simulink model "Generator_Testrig"  (R2019b)
settings: Solver=ode23t  StartTime=0.0  StopTime=15  MaxStep=0.01  RelTol=1e-5  EnableMultiTasking=on
PreLoadFcn:
  | load Generator_Test_DATA
PostLoadFcn:
  | warning off ne_sli:simulator:input:FilteredInputs
undefined symbols (not defined in the file): radps2rpm, WT_Params
libraries: powerlib x6, fl_lib x6, nesl_utility x4, Generator_Lib x1, powerlib_extras x1, Geartrain_Lib x1, simulink x1
Description:
  | Copyright 2009-2017 The MathWorks, Inc. MathWorks, Inc.
settings Model: Creator=smiller  LastModifiedBy=bhisma
settings DataIOCC: LimitDataPoints=on  SaveFormat=Array  SignalLoggingSaveFormat=ModelDataLogs  ReturnWorkspaceOutputs=off
settings OptimizationCC: ExpressionDepthLimit=2147483647  LifeSpan=inf
settings DebuggingCC: UnderspecifiedInitializationDetection=Classic  MergeDetectMultiDrivingBlocksExec=none  SolverPrmCheckMsg=warning  FcnCallInpInsideContextMsg=warning  AllowSymbolicDim=off  StateNameClashWarn=warning  SFUnexpectedBacktrackingDiag=warning  SFNoUnconditionalDefaultTransitionDiag=warning  SFExecutionAtInitializationDiag=none  ArithmeticOperatorsInVariantConditions=warning
settings HardwareCC: ProdBitPerPointer=32  ProdBitPerSizeT=32  ProdBitPerPtrDiffT=32  ProdLargestAtomicFloat=None  ProdIntDivRoundTo=Undefined  ProdEndianess=Unspecified  ProdWordSize=32  ProdHWDeviceType=32-bit Generic
settings ModelReferenceCC: PropagateSignalLabelsOutOfModel=off
settings SFSimCC: SimUseLocalCustomCode=off  CustomCodeUndefinedFunction=UseInterfaceOnly
settings RTWCC: RTWUseLocalCustomCode=off
settings CodeAppCC: StateflowObjectComments=on
settings GRTTargetCC: TargetLangStandard=C89/C90 (ANSI)  GeneratePreprocessorConditionals=Disable all  CombineOutputUpdateFcns=off  GRTInterface=on
settings ConfigComp: CovMetricSettings=dw  CovHtmlReporting=on  CovSaveCumulativeToWorkspaceVar=on  CovSaveSingleToWorkspaceVar=on  CovExternalEMLEnable=off  CovSFcnEnable=off
settings SimscapeCC: SimscapeNormalizeSystem=off  SimscapeNominalValues="[{\"value\":\"10\",\"unit\":\"V\"},{\"value\":\"1\",\"unit\":\"A\"},{\"value\":\"10\",\"unit\":\"N*m\"},{\"value\":\"10\",\"unit\":\"bar\"},{\"value\":\"100\",\"unit\":\"kJ/kg\"},{\"value\":\"1\",\"unit\":\"kW\"},{\"value\":\"300\",\"unit\":\"K\"},{\"value\":\"100\",\"unit\":\"cm^3/s\"},{\"value\":\"1\",\"unit\":\"kN\"},{\"value\":\"1\",\"unit\":\"g/cm^3\"},{\"value\":\"1\",\"unit\":\"l\"},{\"value\":\"1\",\"unit\":\"cm^2\"},{\"value\":\"60\",\"unit\":\"Hz\"}]"

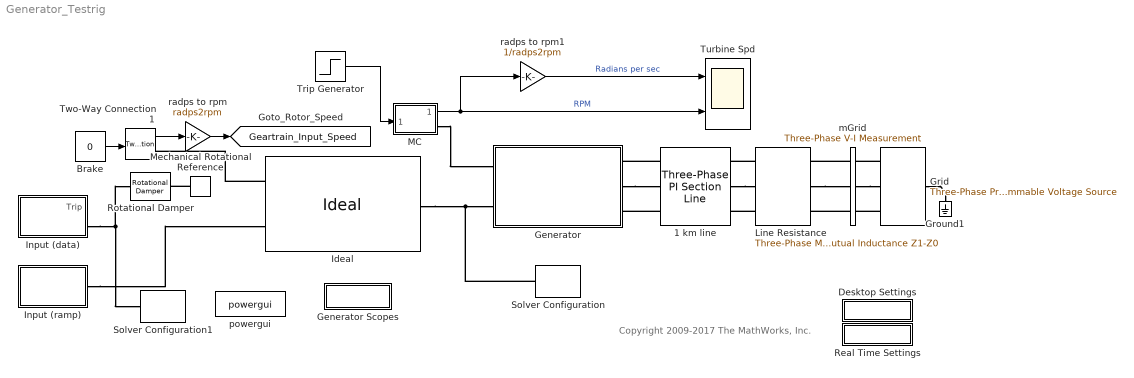
== system Generator_Testrig ==
  note: Copyright 2009-2017 The MathWorks, Inc.
  "1 km line " : powerlib/Elements/Three-Phase PI Section Line  LConnTagsString=a|b|c  RConnTagsString=A|B|C  Frequency=WT_Params.Grid.frequency  Resistances=[0.1153 0.413]  Inductances=[1.05e-3 3.32e-3]  Capacitances=[11.33e-009 5.01e-009]  Length=1
      settings: SourceProductName=Simscape Electrical
  Brake : Constant  Value=0
  Desktop Settings : Subsystem
      settings: OpenFcn=|
      | set_param(bdroot,'Solver','ODE23t','MaxStep','0.01');
      | 
      | tvar_solverBlock = find_system(bdroot, 'SubClassName', 'solver');
      | 
      | for i=1:size(tvar_solverBlock,1)
      | 
      | set_param(char(tvar_solverBlock(i)), 'UseLocalSolver','off','DoFixedCost','off');
      | end
      | 
      | clear tvar_solverBlock
      mask Display: disp('Desktop')
  Generator : Subsystem  BlockChoice=Full
      link override Full/B_Gen/Model/VI/Ia: GotoTag=tpdea4285c_d746_48d3_8c95_fd37d852a013_Ia
      link override Full/B_Gen/Model/VI/Ib: GotoTag=tpdea4285c_d746_48d3_8c95_fd37d852a013_Ib
      link override Full/B_Gen/Model/VI/Ic: GotoTag=tpdea4285c_d746_48d3_8c95_fd37d852a013_Ic
      link override Full/B_Gen/Model/VI/Va: GotoTag=tpdea4285c_d746_48d3_8c95_fd37d852a013_Va
      link override Full/B_Gen/Model/VI/Vb: GotoTag=tpdea4285c_d746_48d3_8c95_fd37d852a013_Vb
      link override Full/B_Gen/Model/VI/Vc: GotoTag=tpdea4285c_d746_48d3_8c95_fd37d852a013_Vc
      settings: AttributesFormatString=%<BlockChoice>  TemplateBlock=Generator_Lib/Generator  MemberBlocks=Full,Simple
      mask Display: disp(' ')
  Generator Scopes : Subsystem  AncestorBlock=Generator_Lib/Generator Scopes
  Grid : powerlib/Electrical Sources/Three-Phase Programmable Voltage Source  PositiveSequence=[WT_Params.Grid.voltage 0 WT_Params.Grid.frequency]  VariationEntity=None  VariationType=Table of time-amplitude pairs  VariationTypeAlt=Step  VariationStep=-0.15  VariationRate=10  VariationMagnitude=0.3  VariationFrequency=2  VariationTiming=[5 5.5]  VariationPhaseA=off  Amplitudes="[1.0  0.5  1.0 ]"  TimeValues="[0  10  10.1]"  HarmonicGeneration=off  HarmonicA=[1 -0.1 0 1]  HarmonicB=[2 0.15 35 2]  Timing="[5  5.5]"  BusType=swing  Pref=0  Qref=0  Qmin=-inf  Qmax=inf
      settings: SourceProductName=Simscape Electrical
  Ground1 : powerlib/Elements/Ground  LConnTagsString=a
      settings: SourceProductName=Simscape Electrical
  Ideal : Geartrain_Lib/Ideal  SystemSampleTime=-1
  Input (data) : Subsystem
  Input (ramp) : Subsystem  mask{start_speed=0, final_speed=14.3004, start_time=3, stop_time=10}
      mask prompts: start_speed "Start speed (rpm)"; final_speed "Final speed (rpm)"; start_time "Ramp start time"; stop_time "Ramp stop time"
  Line Resistance : powerlib/Elements/Three-Phase Mutual Inductance Z1-Z0  LConnTagsString=a|b|c  RConnTagsString=A|B|C  PositiveSequence="[0.1  1.0/(2*pi*60)]*WT_Params.Grid.voltage^2/2500e6"  ZeroSequence="[0.3  3.0/(2*pi*60)]*WT_Params.Grid.voltage^2/2500e6"
      settings: SourceProductName=Simscape Electrical  SourceProductBaseCode=PS
  MC : Subsystem
  Mechanical Rotational Reference : fl_lib/Mechanical/Rotational Elements/Mechanical Rotational Reference
  Real Time Settings : Subsystem
      settings: OpenFcn=|
      | tvar_Nonlinear_Iterations = '3';
      | tvar_StepSize = '0.001';
      | %tvar_LocalSolver='NE_TRAPEZOIDAL_ADVANCER';
      | tvar_LocalSolver='NE_BACKWARD_EULER_ADVANCER';
      | set_param(bdroot,'Solver','ode3','FixedStep','auto');
      | tvar_solverBlock = find_system(bdroot, 'SubClassName', 'solver');
      | for i=1:size(tvar_solverBlock,1)
      |     set_param(char(tvar_solverBlock(i)), 'UseLocalSolver','on','DoFixedCost','on','MaxNonlinIter',tvar_Nonlinear_Iterations,'LocalSolverChoice',tvar_LocalSolver,'LocalSolverSampleTime',tvar_StepSize);
      | end
      | clear tvar_Nonlinear_Iterations tvar_StepSize tvar_LocalSolver tvar_solverBlock
      mask Display: disp('Real Time')
  Rotational Damper : fl_lib/Mechanical/Rotational Elements/Rotational Damper  D=0.001 N*m/(rad/s)  w_specify=off  w_priority=High  w=0 rad/s  w_nominal_specify=off  w_nominal_unit=rad/s  w_nominal_value=1  t_specify=off  t_priority=High  t=0 N*m  t_nominal_specify=off  t_nominal_unit=N*m  t_nominal_value=1
  Solver Configuration : nesl_utility/Solver Configuration  PhysicalDomain=network_engine_domain  SubClassName=solver  LeftPortType=input  RightPortType=generic  Tones=[]  Harmonics=[]  SimulateNoise=off  Profile=off  UseLocalSampling=off  EnableSwitchedLinearOptims=on  FrequencyDomain=off  UseCCode=off  RelTol=0.001  AbsTol=1e-06  MinStep=1e-09  ToWorkspace=off  RevertToSquareIcSolve=off  NumHomotopyIterations=100  PhasorMode=off  PhasorModeNumHarmonics=1  DoDC=off  ResidualTolerance=1e-9  UseLocalSolver=off  LocalSolverChoice=NE_BACKWARD_EULER_ADVANCER  LocalSolverSampleTime=0.001  DoFixedCost=off  MaxNonlinIter=3  MaxModeIter=2  LinearAlgebra=Sparse  EquationFormulation=NE_TIME_EF  DelaysMemoryBudget=1024  AutomaticFiltering=on  FilteringTimeConstant=0.001  PartitionStorageMethod=AS_NEEDED  PartitionMemoryBudget=1024  PartitionMethod=FAST
  Solver Configuration1 : nesl_utility/Solver Configuration  PhysicalDomain=network_engine_domain  SubClassName=solver  LeftPortType=input  RightPortType=generic  Tones=[]  Harmonics=[]  SimulateNoise=off  Profile=off  UseLocalSampling=off  EnableSwitchedLinearOptims=on  FrequencyDomain=off  UseCCode=off  RelTol=0.001  AbsTol=1e-06  MinStep=1e-09  ToWorkspace=off  RevertToSquareIcSolve=off  NumHomotopyIterations=100  PhasorMode=off  PhasorModeNumHarmonics=1  DoDC=off  ResidualTolerance=1e-9  UseLocalSolver=off  LocalSolverChoice=NE_BACKWARD_EULER_ADVANCER  LocalSolverSampleTime=0.001  DoFixedCost=off  MaxNonlinIter=3  MaxModeIter=2  LinearAlgebra=Sparse  EquationFormulation=NE_TIME_EF  DelaysMemoryBudget=1024  AutomaticFiltering=on  FilteringTimeConstant=0.001  PartitionStorageMethod=AS_NEEDED  PartitionMemoryBudget=1024  PartitionMethod=FAST
  Trip Generator : Step  Time=10  Before=1  After=0  SampleTime=0
  Turbine Spd : Scope  NumInputPorts=2
  Two-Way Connection1 : TwoWayConnection
  mGrid : powerlib/Measurements/Three-Phase V-I Measurement  VoltageMeasurement=phase-to-ground  SetLabelV=on  LabelV=VmGrid  Vpu=on  VpuLL=off  CurrentMeasurement=no  SetLabelI=on  LabelI=ImGrid  Ipu=off  Pbase=1.5e6/0.9  Vbase=25e3  OutputType=Magnitude  PhasorSimulation=on  PSBequivalent=0
      settings: SourceProductName=Simscape Electrical
  powergui : powerlib/powergui  SimulationMode=Phasor  SampleTime=5e-6  frequency=60  Iterations=50  frequencyindice=60  Pbase=100e6  ErrMax=1e-4  UnitsV=kV  UnitsW=MW  buscounter=0  FunctionMessages=off  echomessages=off  EnableUseOfTLC=off  CurrentSourceSwitches=off  DisableSnubberDevices=off  DisableRonSwitches=off  DisableVfSwitches=off  DisplayEquations=off  AutomaticDiscreteSolvers=off  SolverType=Tustin  Interpol=off  ExternalGateDelay=off  methode=off  Ts=0  x0status=blocks  SPID=off  SwTol=0  HookPort=off  NonlinearTolerance=1e-4  nMaxIteration=100  ContinueOnMaxIteration=off  RestoreLinks=warning  ResistiveCurrentMeasurement=off  Frange=[0:2:500]  Ylog=off  Xlog=on  ShowGrid=off  save=off  variable=ZData  structure=0  ZoomFFT=on  StartTime=0.0  cycles=1  DisplayStyle=1  fundamental=60  FreqAxis=off  MaxFrequency=1000  frequencyindicesteady=1  RmsSteady=1  display=off
      settings: SourceProductName=Simscape Electrical
  radps to rpm : Gain  Gain=radps2rpm
  radps to rpm1 : Gain  Gain=1/radps2rpm
  tag scope: Geartrain_Input_Speed=global
  wires:
  MC/1(Speed) -> radps to rpm1/1, Turbine Spd/2  "RPM"
  Two-Way Connection1/1 -> radps to rpm/1
  Brake/1 -> Two-Way Connection1/1
  radps to rpm/1 -> [Geartrain_Input_Speed]
  radps to rpm1/1 -> Turbine Spd/1  "Radians per sec"
  Trip Generator/1 -> MC/1(Trip)
  connections:
  Grid/LConn1 -- Ground1/LConn1
  Line Resistance/RConn1 -- "1 km line "/LConn1
  "1 km line "/LConn2 -- Line Resistance/RConn2
  Line Resistance/RConn3 -- "1 km line "/LConn3
  Grid/RConn1 -- mGrid/LConn1
  mGrid/LConn2 -- Grid/RConn2
  Grid/RConn3 -- mGrid/LConn3
  mGrid/RConn1 -- Line Resistance/LConn1
  Line Resistance/LConn2 -- mGrid/RConn2
  mGrid/RConn3 -- Line Resistance/LConn3
  Ideal/RConn1 -- Solver Configuration/RConn1 -- Generator/LConn2
  "1 km line "/RConn1 -- Generator/RConn1
  Generator/RConn2 -- "1 km line "/RConn2
  "1 km line "/RConn3 -- Generator/RConn3
  MC/RConn1 -- Generator/LConn1
  Ideal/LConn1 -- Two-Way Connection1/RConn1
  Input (data)/RConn1 -- Solver Configuration1/RConn1 -- Rotational Damper/LConn1
  Input (ramp)/LConn1 -- Ideal/LConn2
  Mechanical Rotational Reference/LConn1 -- Rotational Damper/RConn1

== system Generator_Testrig/Desktop Settings ==

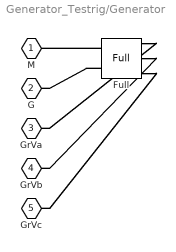
== system Generator_Testrig/Generator ==
  Full : Generator_Lib/Full  SystemSampleTime=-1
  M : PMIOPort  Side=Left
  G : PMIOPort  Port=2  Side=Left
  GrVa : PMIOPort  Port=3  Side=Right
  GrVb : PMIOPort  Port=4  Side=Right
  GrVc : PMIOPort  Port=5  Side=Right
  connections:
  Full/LConn1 -- M/RConn1
  Full/LConn2 -- G/RConn1
  Full/RConn1 -- GrVa/RConn1
  Full/RConn2 -- GrVb/RConn1
  Full/RConn3 -- GrVc/RConn1

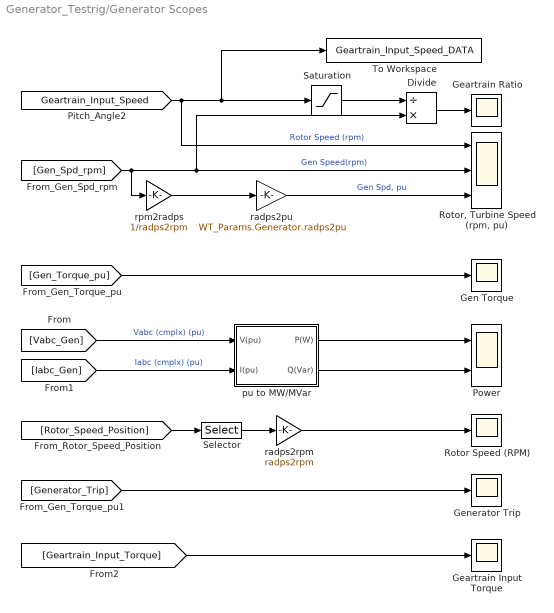
== system Generator_Testrig/Generator Scopes ==
  Divide : Product  Inputs=/*
  Geartrain Input Torque : Scope
  Geartrain Ratio : Scope
  Gen Torque : Scope
  Generator Trip : Scope
  Power : Scope  NumInputPorts=2
  Rotor Speed (RPM) : Scope
  "Rotor, Turbine Speed (rpm, pu)" : Scope  NumInputPorts=3
  Saturation : Saturate  UpperLimit=inf  LowerLimit=eps
  Selector : Selector  InputPortWidth=2  IndexOptions=Index vector (dialog)  Indices=[2]  OutputSizes=1
  To Workspace : ToWorkspace  VariableName=Geartrain_Input_Speed_DATA  SaveFormat=Structure With Time  SampleTime=-1
  pu to MW/MVar : Subsystem
  radps2pu : Gain  Gain=WT_Params.Generator.radps2pu
  radps2rpm : Gain  Gain=radps2rpm
  rpm2radps : Gain  Gain=1/radps2rpm
  wires:
  [Generator_Trip] -> Generator Trip/1
  pu to MW/MVar/2(Q(Var)) -> Power/2
  pu to MW/MVar/1(P(W)) -> Power/1
  [Gen_Torque_pu] -> Gen Torque/1
  [Iabc_Gen] -> pu to MW/MVar/2(I(pu))  "Iabc (cmplx) (pu)"
  [Vabc_Gen] -> pu to MW/MVar/1(V(pu))  "Vabc (cmplx) (pu)"
  [Geartrain_Input_Speed] -> "Rotor, Turbine Speed (rpm, pu)"/1, Saturation/1, To Workspace/1  "Rotor Speed (rpm)"
  radps2pu/1 -> "Rotor, Turbine Speed (rpm, pu)"/3  "Gen Spd, pu"
  rpm2radps/1 -> radps2pu/1
  Divide/1 -> Geartrain Ratio/1
  [Gen_Spd_rpm] -> "Rotor, Turbine Speed (rpm, pu)"/2, Divide/2, rpm2radps/1  "Gen Speed(rpm)"
  [Rotor_Speed_Position] -> Selector/1
  Selector/1 -> radps2rpm/1
  radps2rpm/1 -> Rotor Speed (RPM)/1
  Saturation/1 -> Divide/1
  [Geartrain_Input_Torque] -> Geartrain Input Torque/1

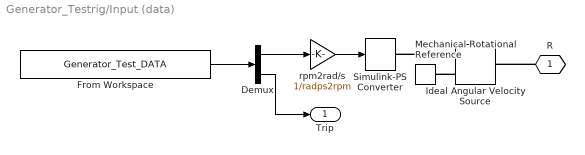
== system Generator_Testrig/Input (data) ==
  Demux : Demux  Outputs=2
  From Workspace : FromWorkspace  VariableName=Generator_Test_DATA  SampleTime=0
  Ideal Angular Velocity Source : fl_lib/Mechanical/Mechanical Sources/Ideal Angular Velocity Source
  Mechanical Rotational Reference : fl_lib/Mechanical/Rotational Elements/Mechanical Rotational Reference
  Simulink-PS Converter : nesl_utility/Simulink-PS Converter  PhysicalDomain=network_engine_domain  SubClassName=ps_input  LeftPortType=input  RightPortType=output  PseudoPeriodic=off  Frequencies=[]  NoiseDistribution=none  NoiseParameters=[]  Unit=1  AffineConversion=off  FilteringAndDerivatives=zero  SimscapeFilterOrder=1  InputFilterTimeConstant=.001  UdotUserProvided=0
  rpm2rad/s : Gain  Gain=1/radps2rpm
  R : PMIOPort  Tag=PMCPort  Side=Right
  Trip : Outport
  wires:
  rpm2rad/s/1 -> Simulink-PS Converter/1
  From Workspace/1 -> Demux/1
  Demux/1 -> rpm2rad/s/1
  Demux/2 -> Trip/1
  connections:
  R/RConn1 -- Ideal Angular Velocity Source/LConn1
  Ideal Angular Velocity Source/RConn1 -- Simulink-PS Converter/RConn1
  Ideal Angular Velocity Source/RConn2 -- Mechanical Rotational Reference/LConn1

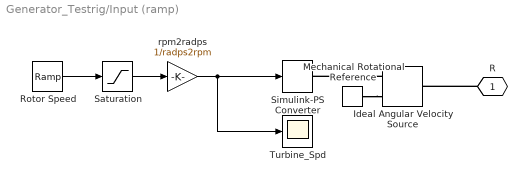
== system Generator_Testrig/Input (ramp) ==
  Ideal Angular Velocity Source : fl_lib/Mechanical/Mechanical Sources/Ideal Angular Velocity Source
  Mechanical Rotational Reference : fl_lib/Mechanical/Rotational Elements/Mechanical Rotational Reference
  Rotor Speed : simulink/Sources/Ramp  slope=(final_speed-start_speed)/(stop_time-start_time)  start=start_time  X0=start_speed
  Saturation : Saturate  UpperLimit=final_speed  LowerLimit=0
  Simulink-PS Converter : nesl_utility/Simulink-PS Converter  PhysicalDomain=network_engine_domain  SubClassName=ps_input  LeftPortType=input  RightPortType=output  PseudoPeriodic=off  Frequencies=[]  NoiseDistribution=none  NoiseParameters=[]  Unit=1  AffineConversion=off  FilteringAndDerivatives=filter  SimscapeFilterOrder=1  InputFilterTimeConstant=WT_Params.Generator.PSLD_Interface_Filter_Coeff  UdotUserProvided=1
  Turbine_Spd : Scope
  rpm2radps : Gain  Gain=1/radps2rpm
  R : PMIOPort  Tag=PMCPort  Side=Left
  wires:
  Rotor Speed/1 -> Saturation/1
  Saturation/1 -> rpm2radps/1
  rpm2radps/1 -> Turbine_Spd/1, Simulink-PS Converter/1
  connections:
  R/RConn1 -- Ideal Angular Velocity Source/LConn1
  Ideal Angular Velocity Source/RConn1 -- Simulink-PS Converter/RConn1
  Mechanical Rotational Reference/LConn1 -- Ideal Angular Velocity Source/RConn2

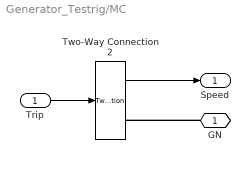
== system Generator_Testrig/MC ==
  Trip : Inport
  Two-Way Connection2 : TwoWayConnection
  GN : PMIOPort  Side=Right
  Speed : Outport
  wires:
  Two-Way Connection2/1 -> Speed/1
  Trip/1 -> Two-Way Connection2/1
  connections:
  GN/RConn1 -- Two-Way Connection2/RConn1

== system Generator_Testrig/Real Time Settings ==

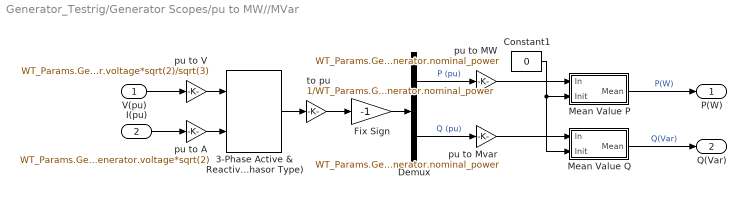
== system Generator_Testrig/Generator Scopes/pu to MW//MVar ==
  V(pu) : Inport
  I(pu) : Inport  Port=2
  3-Phase Active & Reactive Power (Phasor Type) : powerlib_extras/Phasor Library/3-Phase Active & Reactive Power (Phasor Type)
      settings: SourceProductName=Simscape Electrical  SourceProductBaseCode=PS
  Constant1 : Constant  Value=0
  Demux : Demux  Outputs=2
  Fix Sign : Gain  Gain=-1  SaturateOnIntegerOverflow=on  OutDataTypeStr=Inherit: Same as input  ParamDataTypeStr=Inherit: Same as input
  Mean Value P : Subsystem  mask(Mean value){Period=1/WT_Params.Generator.frequency}
      mask prompts: Period "Averaging period (s):"
      mask help: This block uses the running window averaging technique to compute the mean value of the input signal over the specified period.
  Mean Value Q : Subsystem  mask(Mean value){Period=1/WT_Params.Generator.frequency}
      mask prompts: Period "Averaging period (s):"
      mask help: This block uses the running window averaging technique to compute the mean value of the input signal over the specified period.
  pu to A : Gain  Gain=WT_Params.Generator.nominal_power/sqrt(3)/WT_Params.Generator.voltage*sqrt(2)  SaturateOnIntegerOverflow=on  OutDataTypeStr=Inherit: Same as input  ParamDataTypeStr=Inherit: Same as input
  pu to MW : Gain  Gain=WT_Params.Generator.nominal_power  SaturateOnIntegerOverflow=on  OutDataTypeStr=Inherit: Same as input  ParamDataTypeStr=Inherit: Same as input
  pu to Mvar : Gain  Gain=WT_Params.Generator.nominal_power  SaturateOnIntegerOverflow=on  OutDataTypeStr=Inherit: Same as input  ParamDataTypeStr=Inherit: Same as input
  pu to V : Gain  Gain=WT_Params.Generator.voltage*sqrt(2)/sqrt(3)  SaturateOnIntegerOverflow=on  OutDataTypeStr=Inherit: Same as input  ParamDataTypeStr=Inherit: Same as input
  to pu : Gain  Gain=1/WT_Params.Generator.nominal_power  SaturateOnIntegerOverflow=on  OutDataTypeStr=Inherit: Same as input  ParamDataTypeStr=Inherit: Same as input
  P(W) : Outport
  Q(Var) : Outport  Port=2
  wires:
  Mean Value Q/1(Mean) -> Q(Var)/1  "Q(Var)"
  Mean Value P/1(Mean) -> P(W)/1  "P(W)"
  I(pu)/1 -> pu to A/1
  V(pu)/1 -> pu to V/1
  pu to Mvar/1 -> Mean Value Q/1(In)
  Constant1/1 -> Mean Value Q/2(Init), Mean Value P/2(Init)
  pu to MW/1 -> Mean Value P/1(In)
  pu to A/1 -> 3-Phase Active & Reactive Power (Phasor Type)/2
  Fix Sign/1 -> Demux/1
  to pu/1 -> Fix Sign/1
  3-Phase Active & Reactive Power (Phasor Type)/1 -> to pu/1
  pu to V/1 -> 3-Phase Active & Reactive Power (Phasor Type)/1
  Demux/2 -> pu to Mvar/1  "Q (pu)"
  Demux/1 -> pu to MW/1  "P (pu)"

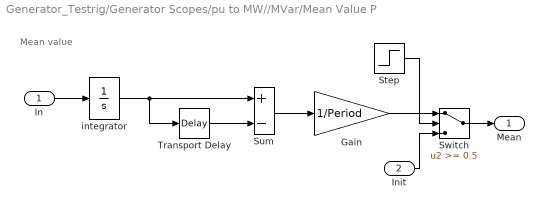
== system Generator_Testrig/Generator Scopes/pu to MW//MVar/Mean Value P ==
  note: Mean value
  In : Inport
  Init : Inport  Port=2
  Gain : Gain  Gain=1/Period  SaturateOnIntegerOverflow=on  OutDataTypeStr=Inherit: Same as input  ParamDataTypeStr=Inherit: Same as input
  Step : Step  Time=Period+eps  SampleTime=0
  Sum : Sum  Inputs=+-  SaturateOnIntegerOverflow=on  InputSameDT=on  OutDataTypeStr=Inherit: Same as first input
  Switch : Switch  Threshold=0.5  SaturateOnIntegerOverflow=on
  Transport Delay : TransportDelay  DelayTime=Period
  integrator : Integrator
  Mean : Outport
  wires:
  Transport Delay/1 -> Sum/2
  integrator/1 -> Transport Delay/1, Sum/1
  In/1 -> integrator/1
  Sum/1 -> Gain/1
  Gain/1 -> Switch/1
  Switch/1 -> Mean/1
  Step/1 -> Switch/2
  Init/1 -> Switch/3

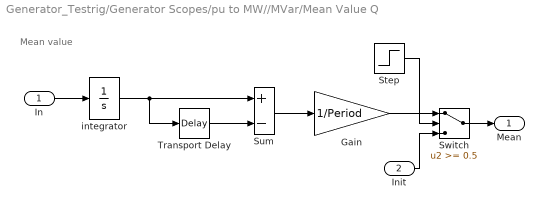
== system Generator_Testrig/Generator Scopes/pu to MW//MVar/Mean Value Q ==
  note: Mean value
  In : Inport
  Init : Inport  Port=2
  Gain : Gain  Gain=1/Period  SaturateOnIntegerOverflow=on  OutDataTypeStr=Inherit: Same as input  ParamDataTypeStr=Inherit: Same as input
  Step : Step  Time=Period+eps  SampleTime=0
  Sum : Sum  Inputs=+-  SaturateOnIntegerOverflow=on  InputSameDT=on  OutDataTypeStr=Inherit: Same as first input
  Switch : Switch  Threshold=0.5  SaturateOnIntegerOverflow=on
  Transport Delay : TransportDelay  DelayTime=Period
  integrator : Integrator
  Mean : Outport
  wires:
  Init/1 -> Switch/3
  Step/1 -> Switch/2
  Switch/1 -> Mean/1
  Gain/1 -> Switch/1
  Sum/1 -> Gain/1
  In/1 -> integrator/1
  integrator/1 -> Sum/1, Transport Delay/1
  Transport Delay/1 -> Sum/2
